simulink model "RLC71"  (R2023a)
settings: Solver=VariableStepAuto  StartTime=0.0  StopTime=1  RelTol=1e-3
libraries: spsIGBTDiodeLib x6, simulink x1, spsDCVoltageSourceLib x1, spsGroundLib x1, spsThreePhaseParallelRLCBranchLib x1, spsThreePhaseVIMeasurementLib x1, spspowerguiLib x1
settings Model: Creator=Asus  LastModifiedBy=DC
settings ModelReferenceCC: EnableRefExpFcnMdlSchedulingChecks=on

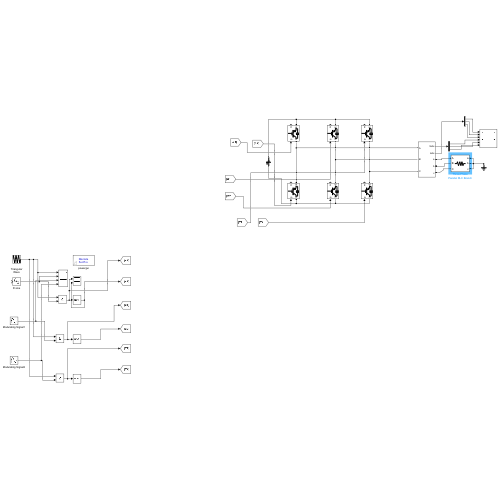
[thumbnail: Simulink's stored preview of the top-level diagram]
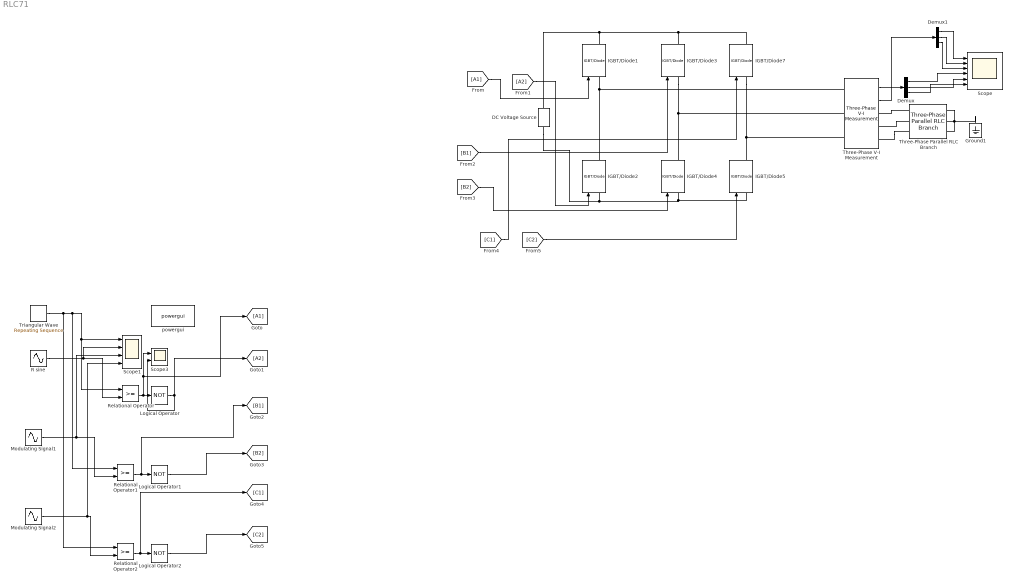
== system RLC71 ==
  " Triangular Wave" : simulink/Sources/Repeating Sequence  rep_seq_t=[0 .25 .5 .75 1]/1050  rep_seq_y=[0 1 0 -1 0]
  DC Voltage Source : spsDCVoltageSourceLib/DC Voltage Source  Amplitude=240  Measurements=None
  Demux : Demux  Outputs=3
  Demux1 : Demux  Outputs=3
  Ground1 : spsGroundLib/Ground  LConnTagsString=a
  IGBT/Diode{1..5,7} (6 alike) : spsIGBTDiodeLib/IGBT//Diode  Ron=1e-2  Rs=1e3  Cs=inf  Measurements=on
  Logical Operator : Logic  Operator=NOT  AllPortsSameDT=off  OutDataTypeStr=boolean
  Logical Operator1 : Logic  Operator=NOT  AllPortsSameDT=off  OutDataTypeStr=boolean
  Logical Operator2 : Logic  Operator=NOT  AllPortsSameDT=off  OutDataTypeStr=boolean
  Modulating Signal1 : Sin  Amplitude=0.4  Frequency=2*pi*50  Phase=2*pi/3  SampleTime=0
  Modulating Signal2 : Sin  Amplitude=0.4  Frequency=2*pi*50  Phase=-2*pi/3  SampleTime=0
  R sine : Sin  TimeSource=Use external signal  Amplitude=0.4  Frequency=2*pi*50  SampleTime=0
  Relational Operator : RelationalOperator  OutDataTypeStr=boolean  RndMeth=Simplest  InputSameDT=off
  Relational Operator1 : RelationalOperator  OutDataTypeStr=boolean  RndMeth=Simplest  InputSameDT=off
  Relational Operator2 : RelationalOperator  OutDataTypeStr=boolean  RndMeth=Simplest  InputSameDT=off
  Scope : Scope  NumInputPorts=6
  Scope1 : Scope  NumInputPorts=4
  Scope3 : Scope  NumInputPorts=2
  Three-Phase Parallel RLC Branch : spsThreePhaseParallelRLCBranchLib/Three-Phase Parallel RLC Branch  LConnTagsString=A|B|C  RConnTagsString=A|B|C  BranchType=R  Resistance=50  Inductance=1e-3  Capacitance=1e-6  Measurements=None
  Three-Phase V-I Measurement : spsThreePhaseVIMeasurementLib/Three-Phase V-I Measurement  VoltageMeasurement=phase-to-ground  SetLabelV=off  LabelV=Vabc  Vpu=off  VpuLL=off  CurrentMeasurement=yes  SetLabelI=off  LabelI=Iabc  Ipu=off  Pbase=100e6  Vbase=500e3  OutputType=Complex  PhasorSimulation=off  PSBequivalent=0
  powergui : spspowerguiLib/powergui  Priority=1  SimulationMode=Discrete  SampleTime=50e-6  frequency=60  Iterations=50  frequencyindice=0  Pbase=100e6  ErrMax=1e-4  UnitsV=kV  UnitsW=MW  buscounter=0  FunctionMessages=off  echomessages=off  EnableUseOfTLC=off  CurrentSourceSwitches=off  DisableSnubberDevices=off  DisableRonSwitches=off  DisableVfSwitches=off  DisplayEquations=off  AutomaticDiscreteSolvers=off  SolverType=Tustin/Backward Euler (TBE)  Interpol=off  ExternalGateDelay=off  methode=off  Ts=100  x0status=blocks  SPID=on  SwTol=0  HookPort=off  NonlinearTolerance=1e-4  nMaxIteration=100  ContinueOnMaxIteration=off  RestoreLinks=warning  ResistiveCurrentMeasurement=off  Frange=[0:2:500]  Ylog=off  Xlog=on  ShowGrid=off  save=off  variable=ZData  structure=0  ZoomFFT=off  StartTime=0.0  cycles=1  DisplayStyle=1  fundamental=60  FreqAxis=off  MaxFrequency=1000  frequencyindicesteady=1  RmsSteady=1  display=off
  wires:
  Relational Operator2/1 -> [C1], Logical Operator2/1
  Relational Operator/1 -> [A1], Scope3/1, Logical Operator/1
  R sine/1 -> Scope1/2, Relational Operator/2
  Relational Operator1/1 -> [B1], Logical Operator1/1
  " Triangular Wave"/1 -> Relational Operator2/1, Relational Operator1/1, Scope1/1, Relational Operator/1
  Modulating Signal1/1 -> Scope1/3, Relational Operator1/2
  Logical Operator/1 -> Scope3/2, [A2]
  Modulating Signal2/1 -> Scope1/4, Relational Operator2/2
  [B1] -> IGBT/Diode3/1
  [C1] -> IGBT/Diode7/1
  [C2] -> IGBT/Diode5/1
  [B2] -> IGBT/Diode4/1
  [A2] -> IGBT/Diode2/1
  [A1] -> IGBT/Diode1/1
  Logical Operator1/1 -> [B2]
  Logical Operator2/1 -> [C2]
  Demux1/2 -> Scope/2
  Demux/1 -> Scope/4
  Demux/2 -> Scope/5
  Demux1/1 -> Scope/1
  Demux1/3 -> Scope/3
  Three-Phase V-I Measurement/2 -> Demux1/1
  Three-Phase V-I Measurement/1 -> Demux/1
  Demux/3 -> Scope/6
  connections:
  IGBT/Diode2/LConn1 -- DC Voltage Source/RConn1 -- IGBT/Diode5/LConn1 -- IGBT/Diode4/LConn1
  IGBT/Diode1/RConn1 -- DC Voltage Source/LConn1 -- IGBT/Diode7/RConn1 -- IGBT/Diode3/RConn1
  IGBT/Diode3/LConn1 -- Three-Phase V-I Measurement/LConn2 -- IGBT/Diode4/RConn1
  Three-Phase Parallel RLC Branch/RConn2 -- Three-Phase Parallel RLC Branch/RConn1 -- Ground1/LConn1 -- Three-Phase Parallel RLC Branch/RConn3
  Three-Phase Parallel RLC Branch/LConn1 -- Three-Phase V-I Measurement/RConn1
  Three-Phase Parallel RLC Branch/LConn3 -- Three-Phase V-I Measurement/RConn3
  Three-Phase Parallel RLC Branch/LConn2 -- Three-Phase V-I Measurement/RConn2
  IGBT/Diode7/LConn1 -- IGBT/Diode5/RConn1 -- Three-Phase V-I Measurement/LConn3
  IGBT/Diode2/RConn1 -- Three-Phase V-I Measurement/LConn1 -- IGBT/Diode1/LConn1
